simulink model "idq"  (R2021a)
settings: Solver=VariableStepAuto  StartTime=0.0  StopTime=0.2  FixedStep=1/150000  MaxStep=1e-6
undefined symbols (not defined in the file): in, ou
libraries: neural x105, spsMosfetLib x12, simulink x5, pid_lib x3, spsabctodq0Lib x3, spsFirstOrderFilterLib x2, spsPermanentMagnetSynchronousMachineLib x2, spsCurrentMeasurementLib x2, spsDCVoltageSourceLib x2, spsThreePhaseVIMeasurementLib x2, spsabctoAlphaBetaZeroLib x2, spsSVPWMGenerator2LevelLib x1
(part 4 of 7)

== system idq/NARX Neural Network - Closed Loop1/Layer 1/Delays 1 ==
  "p{1}" : Inport  PortDimensions=4  SampleTime=1e-05
      mask Display: e = 0.06;c1 = [120 230 180]/255;c2 = ([120 230 180]+0)/(256+128);c3 = ([120 230 180]+128)/(256+128);patch([0 1 1 0],[0 0 1 1],c1);patch([0 1 1 1-e 1-e 0+e],[0 0 1 1-e 0+e 0+e],c2);patch([0 0 1 1-e 0+e 0+e],[0 1 1 1-e 1-e 0+e],c3);plot([0 1 1 0 0],[0 0 1 1 0]);
  Delay 1 : UnitDelay  InitialCondition=pi_input_1_delayed_1  SampleTime=1e-05
      mask Display: e = 0.06;c1 = [120 150 230]/255;c2 = ([120 150 230]+0)/383;c3 = ([120 150 230]+128)/383;patch([0 1 1 0],[0 0 1 1],c1);patch([0 1 1 1-e 1-e 0+e],[0 0 1 1-e 0+e 0+e],c2);patch([0 0 1 1-e 0+e 0+e],[0 1 1 1-e 1-e 0+e],c3);plot([0 1 1 0 0],[0 0 1 1 0]);disp('D')
  Delay 10 : UnitDelay  InitialCondition=pi_input_1_delayed_10  SampleTime=1e-05
      mask Display: e = 0.06;c1 = [120 150 230]/255;c2 = ([120 150 230]+0)/383;c3 = ([120 150 230]+128)/383;patch([0 1 1 0],[0 0 1 1],c1);patch([0 1 1 1-e 1-e 0+e],[0 0 1 1-e 0+e 0+e],c2);patch([0 0 1 1-e 0+e 0+e],[0 1 1 1-e 1-e 0+e],c3);plot([0 1 1 0 0],[0 0 1 1 0]);disp('D')
  Delay 2 : UnitDelay  InitialCondition=pi_input_1_delayed_2  SampleTime=1e-05
      mask Display: e = 0.06;c1 = [120 150 230]/255;c2 = ([120 150 230]+0)/383;c3 = ([120 150 230]+128)/383;patch([0 1 1 0],[0 0 1 1],c1);patch([0 1 1 1-e 1-e 0+e],[0 0 1 1-e 0+e 0+e],c2);patch([0 0 1 1-e 0+e 0+e],[0 1 1 1-e 1-e 0+e],c3);plot([0 1 1 0 0],[0 0 1 1 0]);disp('D')
  Delay 3 : UnitDelay  InitialCondition=pi_input_1_delayed_3  SampleTime=1e-05
      mask Display: e = 0.06;c1 = [120 150 230]/255;c2 = ([120 150 230]+0)/383;c3 = ([120 150 230]+128)/383;patch([0 1 1 0],[0 0 1 1],c1);patch([0 1 1 1-e 1-e 0+e],[0 0 1 1-e 0+e 0+e],c2);patch([0 0 1 1-e 0+e 0+e],[0 1 1 1-e 1-e 0+e],c3);plot([0 1 1 0 0],[0 0 1 1 0]);disp('D')
  Delay 4 : UnitDelay  InitialCondition=pi_input_1_delayed_4  SampleTime=1e-05
      mask Display: e = 0.06;c1 = [120 150 230]/255;c2 = ([120 150 230]+0)/383;c3 = ([120 150 230]+128)/383;patch([0 1 1 0],[0 0 1 1],c1);patch([0 1 1 1-e 1-e 0+e],[0 0 1 1-e 0+e 0+e],c2);patch([0 0 1 1-e 0+e 0+e],[0 1 1 1-e 1-e 0+e],c3);plot([0 1 1 0 0],[0 0 1 1 0]);disp('D')
  Delay 5 : UnitDelay  InitialCondition=pi_input_1_delayed_5  SampleTime=1e-05
      mask Display: e = 0.06;c1 = [120 150 230]/255;c2 = ([120 150 230]+0)/383;c3 = ([120 150 230]+128)/383;patch([0 1 1 0],[0 0 1 1],c1);patch([0 1 1 1-e 1-e 0+e],[0 0 1 1-e 0+e 0+e],c2);patch([0 0 1 1-e 0+e 0+e],[0 1 1 1-e 1-e 0+e],c3);plot([0 1 1 0 0],[0 0 1 1 0]);disp('D')
  Delay 6 : UnitDelay  InitialCondition=pi_input_1_delayed_6  SampleTime=1e-05
      mask Display: e = 0.06;c1 = [120 150 230]/255;c2 = ([120 150 230]+0)/383;c3 = ([120 150 230]+128)/383;patch([0 1 1 0],[0 0 1 1],c1);patch([0 1 1 1-e 1-e 0+e],[0 0 1 1-e 0+e 0+e],c2);patch([0 0 1 1-e 0+e 0+e],[0 1 1 1-e 1-e 0+e],c3);plot([0 1 1 0 0],[0 0 1 1 0]);disp('D')
  Delay 7 : UnitDelay  InitialCondition=pi_input_1_delayed_7  SampleTime=1e-05
      mask Display: e = 0.06;c1 = [120 150 230]/255;c2 = ([120 150 230]+0)/383;c3 = ([120 150 230]+128)/383;patch([0 1 1 0],[0 0 1 1],c1);patch([0 1 1 1-e 1-e 0+e],[0 0 1 1-e 0+e 0+e],c2);patch([0 0 1 1-e 0+e 0+e],[0 1 1 1-e 1-e 0+e],c3);plot([0 1 1 0 0],[0 0 1 1 0]);disp('D')
  Delay 8 : UnitDelay  InitialCondition=pi_input_1_delayed_8  SampleTime=1e-05
      mask Display: e = 0.06;c1 = [120 150 230]/255;c2 = ([120 150 230]+0)/383;c3 = ([120 150 230]+128)/383;patch([0 1 1 0],[0 0 1 1],c1);patch([0 1 1 1-e 1-e 0+e],[0 0 1 1-e 0+e 0+e],c2);patch([0 0 1 1-e 0+e 0+e],[0 1 1 1-e 1-e 0+e],c3);plot([0 1 1 0 0],[0 0 1 1 0]);disp('D')
  Delay 9 : UnitDelay  InitialCondition=pi_input_1_delayed_9  SampleTime=1e-05
      mask Display: e = 0.06;c1 = [120 150 230]/255;c2 = ([120 150 230]+0)/383;c3 = ([120 150 230]+128)/383;patch([0 1 1 0],[0 0 1 1],c1);patch([0 1 1 1-e 1-e 0+e],[0 0 1 1-e 0+e 0+e],c2);patch([0 0 1 1-e 0+e 0+e],[0 1 1 1-e 1-e 0+e],c3);plot([0 1 1 0 0],[0 0 1 1 0]);disp('D')
  mux : Mux  Inputs=10
      mask Display: e = 0.06;c1 = [120 150 230]/255;c2 = ([120 150 230]+0)/383;c3 = ([120 150 230]+128)/383;patch([0 1 1 0],[0 0 1 1],c1);patch([0 1 1 1-e 1-e 0+e],[0 0 1 1-e 0+e 0+e],c2);patch([0 0 1 1-e 0+e 0+e],[0 1 1 1-e 1-e 0+e],c3);plot([0 1 1 0 0],[0 0 1 1 0]);disp('Mux')
  "pd{1,1}" : Outport
      mask Display: e = 0.06;c1 = [120 230 180]/255;c2 = ([120 230 180]+0)/(256+128);c3 = ([120 230 180]+128)/(256+128);patch([0 1 1 0],[0 0 1 1],c1);patch([0 1 1 1-e 1-e 0+e],[0 0 1 1-e 0+e 0+e],c2);patch([0 0 1 1-e 0+e 0+e],[0 1 1 1-e 1-e 0+e],c3);plot([0 1 1 0 0],[0 0 1 1 0]);
  wires:
  "p{1}"/1 -> Delay 1/1
  Delay 1/1 -> Delay 2/1, mux/1
  Delay 2/1 -> Delay 3/1, mux/2
  Delay 3/1 -> Delay 4/1, mux/3
  Delay 4/1 -> Delay 5/1, mux/4
  Delay 5/1 -> Delay 6/1, mux/5
  Delay 6/1 -> Delay 7/1, mux/6
  Delay 7/1 -> Delay 8/1, mux/7
  Delay 8/1 -> Delay 9/1, mux/8
  Delay 9/1 -> Delay 10/1, mux/9
  Delay 10/1 -> mux/10
  mux/1 -> "pd{1,1}"/1

== system idq/NARX Neural Network - Closed Loop1/Layer 1/Delays 2 ==
  "p{1}" : Inport  PortDimensions=1  SampleTime=1e-05
      mask Display: e = 0.06;c1 = [120 230 180]/255;c2 = ([120 230 180]+0)/(256+128);c3 = ([120 230 180]+128)/(256+128);patch([0 1 1 0],[0 0 1 1],c1);patch([0 1 1 1-e 1-e 0+e],[0 0 1 1-e 0+e 0+e],c2);patch([0 0 1 1-e 0+e 0+e],[0 1 1 1-e 1-e 0+e],c3);plot([0 1 1 0 0],[0 0 1 1 0]);
  Delay 1 : UnitDelay  InitialCondition=ai_layer_2_delayed_1  SampleTime=1e-05
      mask Display: e = 0.06;c1 = [120 150 230]/255;c2 = ([120 150 230]+0)/383;c3 = ([120 150 230]+128)/383;patch([0 1 1 0],[0 0 1 1],c1);patch([0 1 1 1-e 1-e 0+e],[0 0 1 1-e 0+e 0+e],c2);patch([0 0 1 1-e 0+e 0+e],[0 1 1 1-e 1-e 0+e],c3);plot([0 1 1 0 0],[0 0 1 1 0]);disp('D')
  Delay 10 : UnitDelay  InitialCondition=ai_layer_2_delayed_10  SampleTime=1e-05
      mask Display: e = 0.06;c1 = [120 150 230]/255;c2 = ([120 150 230]+0)/383;c3 = ([120 150 230]+128)/383;patch([0 1 1 0],[0 0 1 1],c1);patch([0 1 1 1-e 1-e 0+e],[0 0 1 1-e 0+e 0+e],c2);patch([0 0 1 1-e 0+e 0+e],[0 1 1 1-e 1-e 0+e],c3);plot([0 1 1 0 0],[0 0 1 1 0]);disp('D')
  Delay 2 : UnitDelay  InitialCondition=ai_layer_2_delayed_2  SampleTime=1e-05
      mask Display: e = 0.06;c1 = [120 150 230]/255;c2 = ([120 150 230]+0)/383;c3 = ([120 150 230]+128)/383;patch([0 1 1 0],[0 0 1 1],c1);patch([0 1 1 1-e 1-e 0+e],[0 0 1 1-e 0+e 0+e],c2);patch([0 0 1 1-e 0+e 0+e],[0 1 1 1-e 1-e 0+e],c3);plot([0 1 1 0 0],[0 0 1 1 0]);disp('D')
  Delay 3 : UnitDelay  InitialCondition=ai_layer_2_delayed_3  SampleTime=1e-05
      mask Display: e = 0.06;c1 = [120 150 230]/255;c2 = ([120 150 230]+0)/383;c3 = ([120 150 230]+128)/383;patch([0 1 1 0],[0 0 1 1],c1);patch([0 1 1 1-e 1-e 0+e],[0 0 1 1-e 0+e 0+e],c2);patch([0 0 1 1-e 0+e 0+e],[0 1 1 1-e 1-e 0+e],c3);plot([0 1 1 0 0],[0 0 1 1 0]);disp('D')
  Delay 4 : UnitDelay  InitialCondition=ai_layer_2_delayed_4  SampleTime=1e-05
      mask Display: e = 0.06;c1 = [120 150 230]/255;c2 = ([120 150 230]+0)/383;c3 = ([120 150 230]+128)/383;patch([0 1 1 0],[0 0 1 1],c1);patch([0 1 1 1-e 1-e 0+e],[0 0 1 1-e 0+e 0+e],c2);patch([0 0 1 1-e 0+e 0+e],[0 1 1 1-e 1-e 0+e],c3);plot([0 1 1 0 0],[0 0 1 1 0]);disp('D')
  Delay 5 : UnitDelay  InitialCondition=ai_layer_2_delayed_5  SampleTime=1e-05
      mask Display: e = 0.06;c1 = [120 150 230]/255;c2 = ([120 150 230]+0)/383;c3 = ([120 150 230]+128)/383;patch([0 1 1 0],[0 0 1 1],c1);patch([0 1 1 1-e 1-e 0+e],[0 0 1 1-e 0+e 0+e],c2);patch([0 0 1 1-e 0+e 0+e],[0 1 1 1-e 1-e 0+e],c3);plot([0 1 1 0 0],[0 0 1 1 0]);disp('D')
  Delay 6 : UnitDelay  InitialCondition=ai_layer_2_delayed_6  SampleTime=1e-05
      mask Display: e = 0.06;c1 = [120 150 230]/255;c2 = ([120 150 230]+0)/383;c3 = ([120 150 230]+128)/383;patch([0 1 1 0],[0 0 1 1],c1);patch([0 1 1 1-e 1-e 0+e],[0 0 1 1-e 0+e 0+e],c2);patch([0 0 1 1-e 0+e 0+e],[0 1 1 1-e 1-e 0+e],c3);plot([0 1 1 0 0],[0 0 1 1 0]);disp('D')
  Delay 7 : UnitDelay  InitialCondition=ai_layer_2_delayed_7  SampleTime=1e-05
      mask Display: e = 0.06;c1 = [120 150 230]/255;c2 = ([120 150 230]+0)/383;c3 = ([120 150 230]+128)/383;patch([0 1 1 0],[0 0 1 1],c1);patch([0 1 1 1-e 1-e 0+e],[0 0 1 1-e 0+e 0+e],c2);patch([0 0 1 1-e 0+e 0+e],[0 1 1 1-e 1-e 0+e],c3);plot([0 1 1 0 0],[0 0 1 1 0]);disp('D')
  Delay 8 : UnitDelay  InitialCondition=ai_layer_2_delayed_8  SampleTime=1e-05
      mask Display: e = 0.06;c1 = [120 150 230]/255;c2 = ([120 150 230]+0)/383;c3 = ([120 150 230]+128)/383;patch([0 1 1 0],[0 0 1 1],c1);patch([0 1 1 1-e 1-e 0+e],[0 0 1 1-e 0+e 0+e],c2);patch([0 0 1 1-e 0+e 0+e],[0 1 1 1-e 1-e 0+e],c3);plot([0 1 1 0 0],[0 0 1 1 0]);disp('D')
  Delay 9 : UnitDelay  InitialCondition=ai_layer_2_delayed_9  SampleTime=1e-05
      mask Display: e = 0.06;c1 = [120 150 230]/255;c2 = ([120 150 230]+0)/383;c3 = ([120 150 230]+128)/383;patch([0 1 1 0],[0 0 1 1],c1);patch([0 1 1 1-e 1-e 0+e],[0 0 1 1-e 0+e 0+e],c2);patch([0 0 1 1-e 0+e 0+e],[0 1 1 1-e 1-e 0+e],c3);plot([0 1 1 0 0],[0 0 1 1 0]);disp('D')
  mux : Mux  Inputs=10
      mask Display: e = 0.06;c1 = [120 150 230]/255;c2 = ([120 150 230]+0)/383;c3 = ([120 150 230]+128)/383;patch([0 1 1 0],[0 0 1 1],c1);patch([0 1 1 1-e 1-e 0+e],[0 0 1 1-e 0+e 0+e],c2);patch([0 0 1 1-e 0+e 0+e],[0 1 1 1-e 1-e 0+e],c3);plot([0 1 1 0 0],[0 0 1 1 0]);disp('Mux')
  "pd{1,2}" : Outport
      mask Display: e = 0.06;c1 = [120 230 180]/255;c2 = ([120 230 180]+0)/(256+128);c3 = ([120 230 180]+128)/(256+128);patch([0 1 1 0],[0 0 1 1],c1);patch([0 1 1 1-e 1-e 0+e],[0 0 1 1-e 0+e 0+e],c2);patch([0 0 1 1-e 0+e 0+e],[0 1 1 1-e 1-e 0+e],c3);plot([0 1 1 0 0],[0 0 1 1 0]);
  wires:
  "p{1}"/1 -> Delay 1/1
  Delay 1/1 -> Delay 2/1, mux/1
  Delay 2/1 -> Delay 3/1, mux/2
  Delay 3/1 -> Delay 4/1, mux/3
  Delay 4/1 -> Delay 5/1, mux/4
  Delay 5/1 -> Delay 6/1, mux/5
  Delay 6/1 -> Delay 7/1, mux/6
  Delay 7/1 -> Delay 8/1, mux/7
  Delay 8/1 -> Delay 9/1, mux/8
  Delay 9/1 -> Delay 10/1, mux/9
  Delay 10/1 -> mux/10
  mux/1 -> "pd{1,2}"/1

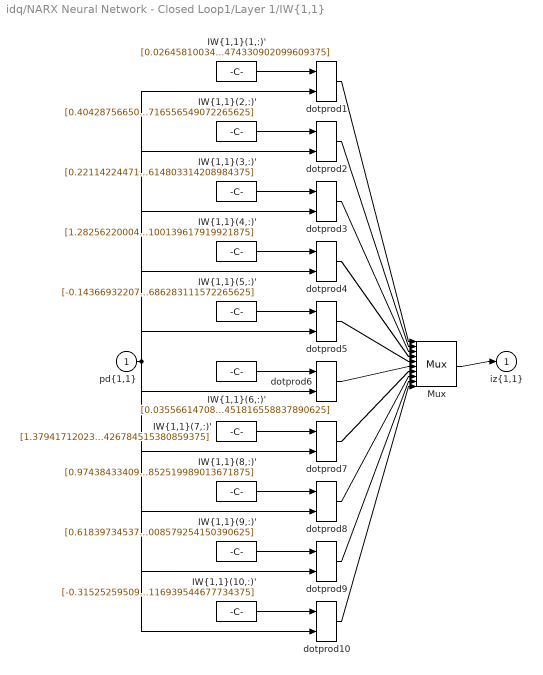
== system idq/NARX Neural Network - Closed Loop1/Layer 1/IW{1,1} ==
  "pd{1,1}" : Inport  PortDimensions=40  SampleTime=1e-05
      mask Display: e = 0.06;c1 = [120 230 180]/255;c2 = ([120 230 180]+0)/(256+128);c3 = ([120 230 180]+128)/(256+128);patch([0 1 1 0],[0 0 1 1],c1);patch([0 1 1 1-e 1-e 0+e],[0 0 1 1-e 0+e 0+e],c2);patch([0 0 1 1-e 0+e 0+e],[0 1 1 1-e 1-e 0+e],c3);plot([0 1 1 0 0],[0 0 1 1 0]);
  "IW{1,1}(1,:)'" : Constant  Value=[0.0264581003444631403243025857818793156184256076812744140625;-0.155011872361149716237349593939143233001232147216796875;0.2800450015320554708608824512339197099208831787109375;-0.035999332393767770332804190047681913711130619049072265625;-0.0231031095312188294865762827612343244254589080810546875;-0.01084188405027063963059763551655123592354357242584228515625;0.2257599227818586073990303475511609576642513275146484375;-0.01362265239200942390507265145060955546796321868896484375;0.0032402507072451232177090485464532321202568709850311279296875;0.0441032571786067195684921671272604726254940032958984375;0.165701195358703701199232227736501954495906829833984375;0.007809907479812143622777131923839988303370773792266845703125;-0.32247695162340495045327770640142261981964111328125;0.05464320885084562873235114466297090984880924224853515625;0.11734475609666546180864798998300102539360523223876953125;0.022042370696496817183973604414859437383711338043212890625;-0.14779113146788847021895207944908179342746734619140625;-0.04890170810500689413391484094972838647663593292236328125;0.06125385435683612656010410546514322049915790557861328125;0.04759689912071306261420744476708932779729366302490234375;-0.15368472929600895948709649019292555749416351318359375;-0.0281595220718017270888910985604525194503366947174072265625;0.0018987226084477061040234335820287014939822256565093994140625;0.073658755859801861021196600631810724735260009765625;-0.4288729543974467706135555999935604631900787353515625;0.08828076784965165069163361977189197205007076263427734375;-0.050871065802078618833803602683474309742450714111328125;0.0882362530759153440573783200306934304535388946533203125;-0.1793763053182588496081706352924811653792858123779296875;0.07017420686064583523755544547384488396346569061279296875;-0.117282277187744810031944098227540962398052215576171875;0.11202104378384718230687866480366210453212261199951171875;-0.25554474369071378259121729570324532687664031982421875;0.027017848729185854617096396168562932871282100677490234375;-0.1817393554574067149331995096872560679912567138671875;0.1373281770518507693967791283284896053373813629150390625;-0.204404914050620833965155043188133276998996734619140625;-0.0668232496942136877660090021890937350690364837646484375;-0.24882893572699382733759421171271242201328277587890625;0.1701278181676374179343014247933751903474330902099609375]
      mask Display: e = 0.06;c1 = [120 150 230]/255;c2 = ([120 150 230]+0)/383;c3 = ([120 150 230]+128)/383;patch([0 1 1 0],[0 0 1 1],c1);patch([0 1 1 1-e 1-e 0+e],[0 0 1 1-e 0+e 0+e],c2);patch([0 0 1 1-e 0+e 0+e],[0 1 1 1-e 1-e 0+e],c3);plot([0 1 1 0 0],[0 0 1 1 0]);disp('Weights');
  "IW{1,1}(10,:)'" : Constant  Value=[-0.31525259509166925209200371682527475059032440185546875;0.031430264941845940940279291453407495282590389251708984375;0.04300350121840725015065487468746141530573368072509765625;0.104894086313607914906498308482696302235126495361328125;-0.1566655845537998914540622763524879701435565948486328125;-0.0716047747138739698602449834652361460030078887939453125;0.03605058399281184378093456643910030834376811981201171875;0.099112432287408680497975410617073066532611846923828125;-0.0631150029612531915379491920248256064951419830322265625;-0.0043770460200082093871198907208963646553456783294677734375;0.0244605474216665376430146494612927199341356754302978515625;0.09132734885736548680057467208825983107089996337890625;0.207052989213431792858699509451980702579021453857421875;-0.0228252538418006155340744811610420583747327327728271484375;0.0028134491170567327809892699264082693844102323055267333984375;0.0912201671514198952905871919938363134860992431640625;-0.04176167714776944650534318270729272626340389251708984375;0.044189429996556554847142450626051868312060832977294921875;-0.00765293292163178075215856921431623050011694431304931640625;0.07987739077519741270894115814371616579592227935791015625;-0.331119784378241188704805608722381293773651123046875;0.0302182814086223404392850255817393190227448940277099609375;-0.0024997052890350555075238414559635202749632298946380615234375;0.06064491989298048668644014469464309513568878173828125;-0.09372638971693357523573553180540329776704311370849609375;-0.08371495819516942826776784158937516622245311737060546875;-0.0029028284625321628363570081177158499485813081264495849609375;0.0520617771870836854031239226969773881137371063232421875;-0.391090681424232922136496881648781709372997283935546875;-0.00136907171975723072898656340612433268688619136810302734375;0.00956503245403937142621320077751079224981367588043212890625;0.0307965875047167721156871067478277836926281452178955078125;-0.16791018620316766618572046354529447853565216064453125;0.052104895448455000595000541352419531904160976409912109375;0.01218678401046962948839347262719456921331584453582763671875;0.0115547261342168229580895655317362979985773563385009765625;-0.28622811444357931787152438118937425315380096435546875;0.070737838842561184815593833263847045600414276123046875;0.0215860086936635504895054538110343855805695056915283203125;-0.01312540017539457447293127501097842468880116939544677734375]
      mask Display: e = 0.06;c1 = [120 150 230]/255;c2 = ([120 150 230]+0)/383;c3 = ([120 150 230]+128)/383;patch([0 1 1 0],[0 0 1 1],c1);patch([0 1 1 1-e 1-e 0+e],[0 0 1 1-e 0+e 0+e],c2);patch([0 0 1 1-e 0+e 0+e],[0 1 1 1-e 1-e 0+e],c3);plot([0 1 1 0 0],[0 0 1 1 0]);disp('Weights');
  "IW{1,1}(2,:)'" : Constant  Value=[0.404287566502792572453728325854171998798847198486328125;-0.403250328667407564875446723817731253802776336669921875;-0.14999270628009586658890839316882193088531494140625;-0.10364376733671888664023441606332198716700077056884765625;0.2307448742481465198128631755025708116590976715087890625;-0.050437412703318300344346170049902866594493389129638671875;-0.1268057176436730160151711288563092239201068878173828125;-0.0735196425771490191802826075218035839498043060302734375;0.0312264234689138171774391850021856953389942646026611328125;0.025309091997740999768762293342660996131598949432373046875;-0.09863467125859355644212911329304915852844715118408203125;-0.04998643840051801567891942568166996352374553680419921875;0.0006075840790996903280352103848827027832157909870147705078125;0.2392835782778407194282266345908283255994319915771484375;-0.0768766146018567686493128121583140455186367034912109375;-0.03444269992289779314109665619980660267174243927001953125;-0.1219129140038336667206664287732564844191074371337890625;0.2146381724825902337361327454345882870256900787353515625;-0.05051196470921050230007409709287458099424839019775390625;-0.018469912687682756013973772724057198502123355865478515625;-0.039545617926555483301331861412108992226421833038330078125;0.0839823188821113841839860469917766749858856201171875;-0.0261787150990239574077644846283874358050525188446044921875;0.00931515752711300527855176056846175924874842166900634765625;-0.09378701116329817011330050036121974699199199676513671875;0.1352867271855986708306573973459308035671710968017578125;-0.002328895548274922087939042825155411264859139919281005859375;0.03612202944687463446182817961016553454101085662841796875;-0.045450745297773757769288494046122650615870952606201171875;0.10946810546046414902576771055464632809162139892578125;0.01812079419329916396552704327405081130564212799072265625;0.06810342611095783482699772548585315234959125518798828125;0.021846413108170710526412250374050927348434925079345703125;0.039722976835466890233039549684690427966415882110595703125;0.03589736716743642530591529293815256096422672271728515625;0.10879854600166682931927653044112958014011383056640625;0.27192689385129475976299318062956444919109344482421875;-0.0904090904617108337415487540056346915662288665771484375;0.044637242455090216097790545290990849025547504425048828125;0.165454465081222912292702176273451186716556549072265625]
      mask Display: e = 0.06;c1 = [120 150 230]/255;c2 = ([120 150 230]+0)/383;c3 = ([120 150 230]+128)/383;patch([0 1 1 0],[0 0 1 1],c1);patch([0 1 1 1-e 1-e 0+e],[0 0 1 1-e 0+e 0+e],c2);patch([0 0 1 1-e 0+e 0+e],[0 1 1 1-e 1-e 0+e],c3);plot([0 1 1 0 0],[0 0 1 1 0]);disp('Weights');
  "IW{1,1}(3,:)'" : Constant  Value=[0.221142244717192515413017872560885734856128692626953125;-0.93569778660913660583986484198248945176601409912109375;-1.18193435088941267707696169964037835597991943359375;-0.0576548752107831907753876521383062936365604400634765625;-0.083464223785847224679201872277189977467060089111328125;0.2316834866348068400210280515238991938531398773193359375;-0.90330499677291964388814449193887412548065185546875;-0.07798091210921719029780518894767737947404384613037109375;-0.038333916777752129190215413245823583565652370452880859375;0.39234373433914970785707510003703646361827850341796875;-0.6371763488163775246420073017361573874950408935546875;-0.0965804397690620819449947020984836854040622711181640625;0.07228590763652760486923654070778866298496723175048828125;0.233456318481962465938295281375758349895477294921875;-0.377851239329094978902645607377053238451480865478515625;-0.09594709433470365034235527446071500889956951141357421875;0.173287318955856528557291085235192440450191497802734375;-0.06467152694635820708857210092901368625462055206298828125;-0.1208347215062860746659367805477813817560672760009765625;-0.0691736180452788562700305874386685900390148162841796875;0.303046772479661774557513354011462070047855377197265625;0.01972742994564956331426941460449597798287868499755859375;0.12176082911210799053502995548114995472133159637451171875;-0.033168749645479535248515645662337192334234714508056640625;0.003865938247603996520684876969653487321920692920684814453125;0.34681971256624333221907363622449338436126708984375;0.36326053562087057269280876425909809768199920654296875;-0.011798579347776984305173897382701397873461246490478515625;0.148265515962799743210354108668980188667774200439453125;0.057579935576568604116420857508273911662399768829345703125;0.60030762805748205668265882195555604994297027587890625;0.0370669086746271692067722369756666012108325958251953125;0.072827707977203004485744486373732797801494598388671875;0.0954199738374567896226352559096994809806346893310546875;0.83437310038273737600178492357372306287288665771484375;0.0913851205560543833339437469476251862943172454833984375;-0.01373924844856483189203810724166032741777598857879638671875;0.0665529738372798440604327652181382291018962860107421875;1.0682475405566993487127547268755733966827392578125;0.1546512514275143190811689919428317807614803314208984375]
      mask Display: e = 0.06;c1 = [120 150 230]/255;c2 = ([120 150 230]+0)/383;c3 = ([120 150 230]+128)/383;patch([0 1 1 0],[0 0 1 1],c1);patch([0 1 1 1-e 1-e 0+e],[0 0 1 1-e 0+e 0+e],c2);patch([0 0 1 1-e 0+e 0+e],[0 1 1 1-e 1-e 0+e],c3);plot([0 1 1 0 0],[0 0 1 1 0]);disp('Weights');
  "IW{1,1}(4,:)'" : Constant  Value=[1.2825622000457881366486390106729231774806976318359375;0.6402270753918768431134367347112856805324554443359375;0.53364884910127596828743890000623650848865509033203125;0.96199324746704295563404230051673948764801025390625;-0.139261364653506358735057801823131740093231201171875;-0.260514823449439159031015833534183911979198455810546875;0.394949614591090014670271557406522333621978759765625;0.77048498608680071608745265621109865605831146240234375;-0.265109506085548840559340533218346536159515380859375;-0.056944306762786216224991875378691474907100200653076171875;0.26531667436419581473927564729820005595684051513671875;0.5605775243995976264699265811941586434841156005859375;-0.459430370835424095599108795795473270118236541748046875;-0.373647780412811714167986565371393226087093353271484375;0.16332127347459224342429706666735000908374786376953125;0.355512911319332436388407359117991290986537933349609375;0.1961768610027908865678369920715340413153171539306640625;-0.0199481518591114494187710448613870539702475070953369140625;0.030391735428321443868160400825217948295176029205322265625;0.145156359393597778062456882253172807395458221435546875;-0.025821863709085034199741670590810826979577541351318359375;-0.323311266568750033112422670455998741090297698974609375;-0.074091974567163709775030611126567237079143524169921875;-0.06210378401063700037898485106779844500124454498291015625;-0.258294007728911534371718516922555863857269287109375;-0.4337132989973355723378745096852071583271026611328125;-0.1548377192350678666077357092945021577179431915283203125;-0.276005961790680320877555686820414848625659942626953125;0.0853071013728281257737506848570774309337139129638671875;-0.01268666256750173963741001870175750809721648693084716796875;-0.253654816395552595853501998135470785200595855712890625;-0.50749597275972313514813549772952683269977569580078125;0.0974932477928580620840648407465778291225433349609375;-0.00628293356560590855741654792154804454185068607330322265625;-0.34338210644061184506625750145758502185344696044921875;-0.745017980219321085399997173226438462734222412109375;-0.033180049462065312748659806629802915267646312713623046875;-0.109708109101965212150986417327658273279666900634765625;-0.414738719536782818320119758936925791203975677490234375;-0.98713307347126011404014889194513671100139617919921875]
      mask Display: e = 0.06;c1 = [120 150 230]/255;c2 = ([120 150 230]+0)/383;c3 = ([120 150 230]+128)/383;patch([0 1 1 0],[0 0 1 1],c1);patch([0 1 1 1-e 1-e 0+e],[0 0 1 1-e 0+e 0+e],c2);patch([0 0 1 1-e 0+e 0+e],[0 1 1 1-e 1-e 0+e],c3);plot([0 1 1 0 0],[0 0 1 1 0]);disp('Weights');
  "IW{1,1}(5,:)'" : Constant  Value=[-0.1436693220731536657641669307849952019751071929931640625;-0.52115555265366031445495309526450000703334808349609375;0.456837527095214801509115432054386474192142486572265625;0.242177332460095484645279384494642727077007293701171875;-0.038548067158590874903278944429985131137073040008544921875;0.097331656080749284765119000439881347119808197021484375;0.374041633215228319642164933611638844013214111328125;0.185228038407303008394677590331411920487880706787109375;-0.08123835698259425364131658398036961443722248077392578125;0.077775369477721179034546139519079588353633880615234375;0.289649153566691908157082480101962573826313018798828125;0.1292714841253526369957427277768147177994251251220703125;-0.01497618847007181445973866829035614500753581523895263671875;-0.05580311822230864249316795167032978497445583343505859375;0.201764684459868559596174009129754267632961273193359375;0.08309633418715101083051877139951102435588836669921875;-0.0728106788515201219791350695231813006103038787841796875;-0.0938938294456459210390875114171649329364299774169921875;0.11309155542180006348562670837054611183702945709228515625;0.038978398558627336267790042256820015609264373779296875;0.1293630264530249152077345797806628979742527008056640625;-0.130215304673179266270466314381337724626064300537109375;0.01237366003115742026097212402646619011647999286651611328125;0.0036234483096465237329797393073249622830189764499664306640625;0.10966413902600401220066572705036378465592861175537109375;-0.1544650141417591715509161076624877750873565673828125;-0.0915698308528863635924466279902844689786434173583984375;-0.029221939429442504720935147588534164242446422576904296875;0.055667093575187905074574956643118639476597309112548828125;-0.1283673098737740103647553269183845259249210357666015625;-0.197545396603328260454190967720933258533477783203125;-0.062766192488151906214710606946027837693691253662109375;0.01455338426129008065623704482050015940330922603607177734375;0.0210914406915475062531672989507569582201540470123291015625;-0.3105121782189390611250701113021932542324066162109375;-0.10291752901469695957725747348376899026334285736083984375;-0.1895138041201333833907227699455688707530498504638671875;-0.012199939972507234386966956662945449352264404296875;-0.41695785435362575643836180461221374571323394775390625;-0.1456274279498782908692788851112709380686283111572265625]
      mask Display: e = 0.06;c1 = [120 150 230]/255;c2 = ([120 150 230]+0)/383;c3 = ([120 150 230]+128)/383;patch([0 1 1 0],[0 0 1 1],c1);patch([0 1 1 1-e 1-e 0+e],[0 0 1 1-e 0+e 0+e],c2);patch([0 0 1 1-e 0+e 0+e],[0 1 1 1-e 1-e 0+e],c3);plot([0 1 1 0 0],[0 0 1 1 0]);disp('Weights');
  "IW{1,1}(6,:)'" : Constant  Value=[0.035566147080295644478109551300804014317691326141357421875;1.345785589579339358579090912826359272003173828125;-0.402906207477657096749368292876170016825199127197265625;0.6797986720358419887588752317242324352264404296875;0.1369844627955762172977216550862067379057407379150390625;-0.244618091905704992949921461331541649997234344482421875;-0.318939589811643442462951725246966816484928131103515625;0.5468220724001309207551457802765071392059326171875;-0.10129533944925443733620085140501032583415508270263671875;-0.1906079832647604443973676779933157376945018768310546875;-0.224199234750296738649666394849191419780254364013671875;0.400797496245371143164248906032298691570758819580078125;0.194530764469177663844590142616652883589267730712890625;-0.484814007758827714145155596270342357456684112548828125;-0.1335829358782410214434577255815383978188037872314453125;0.273897227163087675361197170786908827722072601318359375;0.08667904927128806946701189417581190355122089385986328125;0.1450573233288394714435298737953417003154754638671875;-0.053656940684528871277070294354416546411812305450439453125;0.10934734467499594712247557026785216294229030609130859375;-0.00066320457097665693434185296695204669958911836147308349609375;-0.17630078494639878083916073592263273894786834716796875;0.041018036895985064693714861050466424785554409027099609375;-0.04562004192104786304273744690362946130335330963134765625;0.1764386046788267992102561265710392035543918609619140625;-0.34122065016222913325094623360200785100460052490234375;0.133543882194234464488857838659896515309810638427734375;-0.1914562069350406459111724188915104605257511138916015625;0.12449080008476608172340860392068861983716487884521484375;0.0713948797367921772494270271636196412146091461181640625;0.219164746054576642375621986502665095031261444091796875;-0.362862091309917644821325666271150112152099609375;0.05680601033967312696315588027573539875447750091552734375;-0.15032042761891550863850852692849002778530120849609375;0.316045041099419943275705691121402196586132049560546875;-0.52882727105184923477310121597838588058948516845703125;0.039591312184570272292294390581446350552141666412353515625;-0.006793897015509945021272120158073448692448437213897705078125;0.4117040028798018003186598434695042669773101806640625;-0.7069369862728311915134327136911451816558837890625]
      mask Display: e = 0.06;c1 = [120 150 230]/255;c2 = ([120 150 230]+0)/383;c3 = ([120 150 230]+128)/383;patch([0 1 1 0],[0 0 1 1],c1);patch([0 1 1 1-e 1-e 0+e],[0 0 1 1-e 0+e 0+e],c2);patch([0 0 1 1-e 0+e 0+e],[0 1 1 1-e 1-e 0+e],c3);plot([0 1 1 0 0],[0 0 1 1 0]);disp('Weights');
  "IW{1,1}(7,:)'" : Constant  Value=[1.3794171202312257573652232167660258710384368896484375;-0.346159581390041548587532815872691571712493896484375;-0.280179859204263859151495807964238338172435760498046875;-0.98385897765413010684909522751695476472377777099609375;-0.2003186301421425452584657023180625401437282562255859375;0.156900467902397144914772297852323390543460845947265625;-0.22906869957036024576524368967511691153049468994140625;-0.78775001312269277153887969689094461500644683837890625;-0.38174267080154777875833360667456872761249542236328125;0.1324864654721847057050609919315320439636707305908203125;-0.16405012415898301281202975587802939116954803466796875;-0.58785346579363562113940133713185787200927734375;-0.167994405456998341374941219328320585191249847412109375;0.176292723392869887799605521649937145411968231201171875;-0.1045829654285750642817021116570685990154743194580078125;-0.37749848443712508139213923641364090144634246826171875;0.082772773035674596098232314034248702228069305419921875;0.1294183070281687275571158579623443074524402618408203125;-0.0503420361205701993867478449828922748565673828125;-0.1504635381740809518813506429069093428552150726318359375;-0.100037971533307568083870364716858603060245513916015625;0.329756241550632267500731131804059259593486785888671875;0.0116518794676253763242801397836956311948597431182861328125;0.0689387221945856054627910225462983362376689910888671875;-0.367657730501671498046789565705694258213043212890625;0.199258844350138686341011862168670631945133209228515625;0.0948296532709312078868180151403066702187061309814453125;0.295389495378936828284821558554540388286113739013671875;0.1463406226896686590510654468744178302586078643798828125;0.168389726960378849351940289125195704400539398193359375;0.1604769393953356104720597841151175089180469512939453125;0.54434379618925288202291312700253911316394805908203125;-0.068339219469893575098495830388856120407581329345703125;-0.000101575569080491513729302965884926379658281803131103515625;0.2459985141047987544649089386439300142228603363037109375;0.80413412753415680622737227167817763984203338623046875;0.062828711586723373638818657127558253705501556396484375;0.0688712031143426106627458693765220232307910919189453125;0.329053990697458498271288362957420758903026580810546875;1.0719995747386759088470853384933434426784515380859375]
      mask Display: e = 0.06;c1 = [120 150 230]/255;c2 = ([120 150 230]+0)/383;c3 = ([120 150 230]+128)/383;patch([0 1 1 0],[0 0 1 1],c1);patch([0 1 1 1-e 1-e 0+e],[0 0 1 1-e 0+e 0+e],c2);patch([0 0 1 1-e 0+e 0+e],[0 1 1 1-e 1-e 0+e],c3);plot([0 1 1 0 0],[0 0 1 1 0]);disp('Weights');
  "IW{1,1}(8,:)'" : Constant  Value=[0.97438433409955849118233572880853898823261260986328125;-0.50390909693759977638904956620535813271999359130859375;1.1406444943419000725981504729134030640125274658203125;0.1935714233930634076141785726576927118003368377685546875;-0.230037626477283596582168456734507344663143157958984375;-0.076736593426837196307843669274006970226764678955078125;0.91019517772409452849302624599658884108066558837890625;0.1321891942940303377174160459617269225418567657470703125;-0.293801308204964806147785338907851837575435638427734375;0.067087200562759463640105650483747012913227081298828125;0.6731804084951900080113773583434522151947021484375;0.06894127180237485941205477502080611884593963623046875;-0.300343618894015562670318786331336013972759246826171875;0.0293728393451675728886840488485177047550678253173828125;0.432317865112309906994170205507543869316577911376953125;0.014196811312635525259562285782521939836442470550537109375;0.10574480566003581494260998852041666395962238311767578125;-0.2305338633778089285630841231977683492004871368408203125;0.1737485146974411531761717242261511273682117462158203125;-0.0102633279302546502609327916388792800717055797576904296875;-0.4540161760713943284173410575021989643573760986328125;0.1341797762717078512650914490222930908203125;-0.0747769471183115097545623939367942512035369873046875;-0.060102155936104163791444676689934567548334598541259765625;-0.34702650629720255270882489639916457235813140869140625;-0.1034035988974625619452041291879140771925449371337890625;-0.326907571920222628225616290364996530115604400634765625;-0.08885647364366595912787971656143781729042530059814453125;-0.0354193541146306800637688638744293712079524993896484375;-0.06495838795744911242646679738754755817353725433349609375;-0.60027914743814958509204871006659232079982757568359375;-0.10432799258671097974993102752705453895032405853271484375;-0.08321176893842792410271869130156119354069232940673828125;-0.1610280895387994071210613356015528552234172821044921875;-0.8744657426783837284034461845294572412967681884765625;-0.10896657652523010495482225223895511589944362640380859375;-0.04725140985798427506470176240327418781816959381103515625;0.00588466871349959362580417376875629997812211513519287109375;-1.1602171879175264823658153545693494379520416259765625;-0.113467461566041094567225400169263593852519989013671875]
      mask Display: e = 0.06;c1 = [120 150 230]/255;c2 = ([120 150 230]+0)/383;c3 = ([120 150 230]+128)/383;patch([0 1 1 0],[0 0 1 1],c1);patch([0 1 1 1-e 1-e 0+e],[0 0 1 1-e 0+e 0+e],c2);patch([0 0 1 1-e 0+e 0+e],[0 1 1 1-e 1-e 0+e],c3);plot([0 1 1 0 0],[0 0 1 1 0]);disp('Weights');
  "IW{1,1}(9,:)'" : Constant  Value=[0.6183973453739375347737450283602811396121978759765625;1.09712775640001058974348779884167015552520751953125;0.5366859997957134087442909731180407106876373291015625;-0.7033911209318663981804320428636856377124786376953125;-0.22148016560278749320644919862388633191585540771484375;-0.0493755413216548089128110632373136468231678009033203125;0.41313742358017491174138058340759016573429107666015625;-0.5750293827005032998300748658948577940464019775390625;-0.14586096829948258513098835464916191995143890380859375;-0.335605340685345365780989368431619368493556976318359375;0.2975482081534004397127546326373703777790069580078125;-0.422489371354158815830004414237919263541698455810546875;-0.318728383934667791610451104133971966803073883056640625;-0.1484889040812145122316678680363111197948455810546875;0.188557831206639547882986107651959173381328582763671875;-0.27562342932120309502153077119146473705768585205078125;0.00792415563835606288900503813010800513438880443572998046875;0.1634749328335560469849241371775860898196697235107421875;0.058922429004700883903300479005338274873793125152587890625;-0.1269568559563718224136863454987178556621074676513671875;-0.1410031922517243907488904142155661247670650482177734375;0.023565755460954129762995989949558861553668975830078125;-0.0561746286176641185239333253775839693844318389892578125;0.032333057226810180129206173660350032150745391845703125;-0.304173061325831051160406559574767015874385833740234375;-0.1393205849683144259554268273859634064137935638427734375;-0.1556257721937459315153517991348053328692913055419921875;0.20408972540137437778895446172100491821765899658203125;-0.08098224483692784136934506022953428328037261962890625;-0.05134656823816539927829438738626777194440364837646484375;-0.263867962261181532301890229064156301319599151611328125;0.38537728736803089635287733472068794071674346923828125;-0.057753154616932013409869028919274569489061832427978515625;0.1476803056217402543293104599797516129910945892333984375;-0.37505050817680862795810980969690717756748199462890625;0.56543857536013664155660762844490818679332733154296875;-0.1054480317913007725305618578204303048551082611083984375;0.047941739282653154929914052218009601347148418426513671875;-0.477021505780948318342638003741740249097347259521484375;0.75796026157484386320817293380969204008579254150390625]
      mask Display: e = 0.06;c1 = [120 150 230]/255;c2 = ([120 150 230]+0)/383;c3 = ([120 150 230]+128)/383;patch([0 1 1 0],[0 0 1 1],c1);patch([0 1 1 1-e 1-e 0+e],[0 0 1 1-e 0+e 0+e],c2);patch([0 0 1 1-e 0+e 0+e],[0 1 1 1-e 1-e 0+e],c3);plot([0 1 1 0 0],[0 0 1 1 0]);disp('Weights');
  Mux : Mux  Inputs=10
      mask Display: e = 0.06;c1 = [120 150 230]/255;c2 = ([120 150 230]+0)/383;c3 = ([120 150 230]+128)/383;patch([0 1 1 0],[0 0 1 1],c1);patch([0 1 1 1-e 1-e 0+e],[0 0 1 1-e 0+e 0+e],c2);patch([0 0 1 1-e 0+e 0+e],[0 1 1 1-e 1-e 0+e],c3);plot([0 1 1 0 0],[0 0 1 1 0]);disp('Mux');
  dotprod{1..10} (10 alike) : neural/Weight Functions/dotprod
  "iz{1,1}" : Outport
      mask Display: e = 0.06;c1 = [120 230 180]/255;c2 = ([120 230 180]+0)/(256+128);c3 = ([120 230 180]+128)/(256+128);patch([0 1 1 0],[0 0 1 1],c1);patch([0 1 1 1-e 1-e 0+e],[0 0 1 1-e 0+e 0+e],c2);patch([0 0 1 1-e 0+e 0+e],[0 1 1 1-e 1-e 0+e],c3);plot([0 1 1 0 0],[0 0 1 1 0]);
  wires:
  "IW{1,1}(1,:)'"/1 -> dotprod1/1
  "pd{1,1}"/1 -> dotprod1/2, dotprod2/2, dotprod3/2, dotprod4/2, dotprod5/2, dotprod6/2, dotprod7/2, dotprod8/2, dotprod9/2, dotprod10/2
  dotprod1/1 -> Mux/1
  "IW{1,1}(2,:)'"/1 -> dotprod2/1
  dotprod2/1 -> Mux/2
  "IW{1,1}(3,:)'"/1 -> dotprod3/1
  dotprod3/1 -> Mux/3
  "IW{1,1}(4,:)'"/1 -> dotprod4/1
  dotprod4/1 -> Mux/4
  "IW{1,1}(5,:)'"/1 -> dotprod5/1
  dotprod5/1 -> Mux/5
  "IW{1,1}(6,:)'"/1 -> dotprod6/1
  dotprod6/1 -> Mux/6
  "IW{1,1}(7,:)'"/1 -> dotprod7/1
  dotprod7/1 -> Mux/7
  "IW{1,1}(8,:)'"/1 -> dotprod8/1
  dotprod8/1 -> Mux/8
  "IW{1,1}(9,:)'"/1 -> dotprod9/1
  dotprod9/1 -> Mux/9
  "IW{1,1}(10,:)'"/1 -> dotprod10/1
  dotprod10/1 -> Mux/10
  Mux/1 -> "iz{1,1}"/1

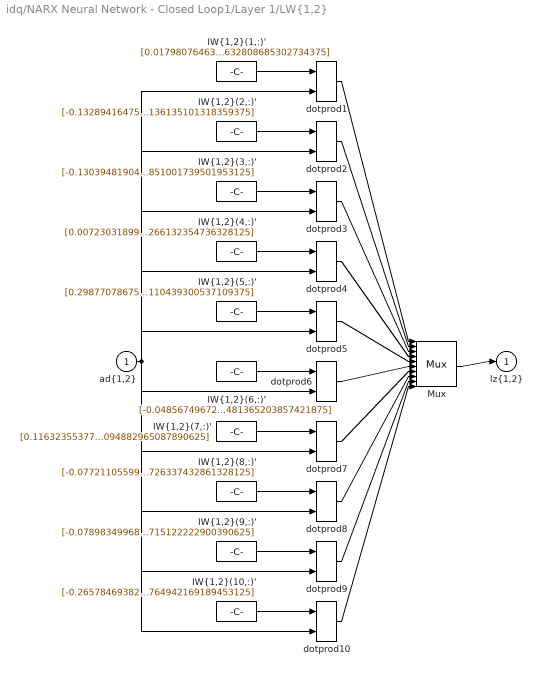
== system idq/NARX Neural Network - Closed Loop1/Layer 1/LW{1,2} ==
  "ad{1,2}" : Inport  PortDimensions=10  SampleTime=1e-05
      mask Display: e = 0.06;c1 = [120 230 180]/255;c2 = ([120 230 180]+0)/(256+128);c3 = ([120 230 180]+128)/(256+128);patch([0 1 1 0],[0 0 1 1],c1);patch([0 1 1 1-e 1-e 0+e],[0 0 1 1-e 0+e 0+e],c2);patch([0 0 1 1-e 0+e 0+e],[0 1 1 1-e 1-e 0+e],c3);plot([0 1 1 0 0],[0 0 1 1 0]);
  "IW{1,2}(1,:)'" : Constant  Value=[0.017980764638247180575714168071499443612992763519287109375;-0.0006884388898641346198059576266814474365673959255218505859375;0.11460027905338464326856495745232678018510341644287109375;0.135802433740163319697558108600787818431854248046875;0.0417070836901971275789691162572125904262065887451171875;0.187143567787656783796279569287435151636600494384765625;0.05116759955733361786567314766216441057622432708740234375;0.13174712189684656404864426804124377667903900146484375;0.109829224742276021498099680684390477836132049560546875;0.09122333474122355789770466572008444927632808685302734375]
      mask Display: e = 0.06;c1 = [120 150 230]/255;c2 = ([120 150 230]+0)/383;c3 = ([120 150 230]+128)/383;patch([0 1 1 0],[0 0 1 1],c1);patch([0 1 1 1-e 1-e 0+e],[0 0 1 1-e 0+e 0+e],c2);patch([0 0 1 1-e 0+e 0+e],[0 1 1 1-e 1-e 0+e],c3);plot([0 1 1 0 0],[0 0 1 1 0]);disp('weights');
  "IW{1,2}(10,:)'" : Constant  Value=[-0.265784693822970485843626420319196768105030059814453125;-0.06802676523812740960739375850607757456600666046142578125;0.2096366117174472964990172840771265327930450439453125;0.2414935230699513379892806597126764245331287384033203125;0.0596576307919906290155864780899719335138797760009765625;0.2040583605379853171513104825862683355808258056640625;0.15905704545408394512406857757014222443103790283203125;0.131804418118469046650176323964842595160007476806640625;0.0786608821238964639466217931840219534933567047119140625;0.09307297361166762261763807373426971025764942169189453125]
      mask Display: e = 0.06;c1 = [120 150 230]/255;c2 = ([120 150 230]+0)/383;c3 = ([120 150 230]+128)/383;patch([0 1 1 0],[0 0 1 1],c1);patch([0 1 1 1-e 1-e 0+e],[0 0 1 1-e 0+e 0+e],c2);patch([0 0 1 1-e 0+e 0+e],[0 1 1 1-e 1-e 0+e],c3);plot([0 1 1 0 0],[0 0 1 1 0]);disp('weights');
  "IW{1,2}(2,:)'" : Constant  Value=[-0.1328941647571120210358230906422249972820281982421875;0.041760579762441608908662971089142956770956516265869140625;0.300977406476627518117084036930464208126068115234375;0.1163565943564725813086369043958256952464580535888671875;-0.135133538483182380485203566422569565474987030029296875;-0.0333122521249077097049706708276062272489070892333984375;0.17687614319344480140472342100110836327075958251953125;0.07608777338393975242514244428093661554157733917236328125;-0.2376845366363752043437074235043837688863277435302734375;0.1128591005765014754214092818074277602136135101318359375]
      mask Display: e = 0.06;c1 = [120 150 230]/255;c2 = ([120 150 230]+0)/383;c3 = ([120 150 230]+128)/383;patch([0 1 1 0],[0 0 1 1],c1);patch([0 1 1 1-e 1-e 0+e],[0 0 1 1-e 0+e 0+e],c2);patch([0 0 1 1-e 0+e 0+e],[0 1 1 1-e 1-e 0+e],c3);plot([0 1 1 0 0],[0 0 1 1 0]);disp('weights');
  "IW{1,2}(3,:)'" : Constant  Value=[-0.130394819045013099501062470153556205332279205322265625;-0.058911588987339780221219598388415761291980743408203125;0.1552891092773753534128644560041720978915691375732421875;0.03923386406291611006036390563167515210807323455810546875;0.039183089224500651515104010513823595829308032989501953125;0.062733761267342369460919826451572589576244354248046875;-0.09111834173013376447780586886437959037721157073974609375;-0.009596242826009397652864407746164943091571331024169921875;-0.00080930608643097769715202272067244848585687577724456787109375;0.0224511326227641479225116682982843485660851001739501953125]
      mask Display: e = 0.06;c1 = [120 150 230]/255;c2 = ([120 150 230]+0)/383;c3 = ([120 150 230]+128)/383;patch([0 1 1 0],[0 0 1 1],c1);patch([0 1 1 1-e 1-e 0+e],[0 0 1 1-e 0+e 0+e],c2);patch([0 0 1 1-e 0+e 0+e],[0 1 1 1-e 1-e 0+e],c3);plot([0 1 1 0 0],[0 0 1 1 0]);disp('weights');
  "IW{1,2}(4,:)'" : Constant  Value=[0.007230318992235625595588199843177790171466767787933349609375;-0.027530049567573565416633840641225106082856655120849609375;0.03931927980824719004449008252777275629341602325439453125;0.1036697490313842340281524911915767006576061248779296875;-0.08800488556615093660440152234514243900775909423828125;-0.0422903883627354648666596403927542269229888916015625;-0.029898614238434172152292234159176587127149105072021484375;-0.04938366367480391538880013513335143215954303741455078125;-0.047652363992253032876078577828593552112579345703125;0.01725052938349276587803871052528847940266132354736328125]
      mask Display: e = 0.06;c1 = [120 150 230]/255;c2 = ([120 150 230]+0)/383;c3 = ([120 150 230]+128)/383;patch([0 1 1 0],[0 0 1 1],c1);patch([0 1 1 1-e 1-e 0+e],[0 0 1 1-e 0+e 0+e],c2);patch([0 0 1 1-e 0+e 0+e],[0 1 1 1-e 1-e 0+e],c3);plot([0 1 1 0 0],[0 0 1 1 0]);disp('weights');
  "IW{1,2}(5,:)'" : Constant  Value=[0.298770786750357952854528775787912309169769287109375;0.1565658388270984302526045439662993885576725006103515625;-0.03629034190341783039368550589642836712300777435302734375;0.02845769943966679205171743660685024224221706390380859375;-0.06332093897910094637548894525025389157235622406005859375;-0.02098231875473570429146974447576212696731090545654296875;0.261792687012228963983062612896901555359363555908203125;-0.2449246884246078781455224770979839377105236053466796875;0.2084687459952666299667356497593573294579982757568359375;-0.1443015658127756173367828296250081621110439300537109375]
      mask Display: e = 0.06;c1 = [120 150 230]/255;c2 = ([120 150 230]+0)/383;c3 = ([120 150 230]+128)/383;patch([0 1 1 0],[0 0 1 1],c1);patch([0 1 1 1-e 1-e 0+e],[0 0 1 1-e 0+e 0+e],c2);patch([0 0 1 1-e 0+e 0+e],[0 1 1 1-e 1-e 0+e],c3);plot([0 1 1 0 0],[0 0 1 1 0]);disp('weights');
  "IW{1,2}(6,:)'" : Constant  Value=[-0.048567496725724357276021692086942493915557861328125;0.049251631944106984140052674092657980509102344512939453125;0.0004353004247698937477506486715128630748949944972991943359375;-0.1621728901973635561528652715423959307372570037841796875;0.155239629465585060597021538342232815921306610107421875;0.043663710965122552731809690840236726216971874237060546875;-0.03155285104801015816367026900479686446487903594970703125;-0.035548053032810687790199466462581767700612545013427734375;0.0575050077603969922446225382373086176812648773193359375;0.027162849826149304544031792829628102481365203857421875]
      mask Display: e = 0.06;c1 = [120 150 230]/255;c2 = ([120 150 230]+0)/383;c3 = ([120 150 230]+128)/383;patch([0 1 1 0],[0 0 1 1],c1);patch([0 1 1 1-e 1-e 0+e],[0 0 1 1-e 0+e 0+e],c2);patch([0 0 1 1-e 0+e 0+e],[0 1 1 1-e 1-e 0+e],c3);plot([0 1 1 0 0],[0 0 1 1 0]);disp('weights');
  "IW{1,2}(7,:)'" : Constant  Value=[0.11632355377996307643773121753838495351374149322509765625;0.02658548085751329115300478633798775263130664825439453125;-0.08825617477343779271325985291696269996464252471923828125;-0.019727139142697337759191356099108816124498844146728515625;-0.059495216370238766800948582158525823615491390228271484375;-0.0342811991043955044400348697308800183236598968505859375;0.0283282351314587503565700643548552761785686016082763671875;-0.0411348273191067814735788488178513944149017333984375;0.026584800562406495083589419436975731514394283294677734375;0.00076116582626404617750726089298041188158094882965087890625]
      mask Display: e = 0.06;c1 = [120 150 230]/255;c2 = ([120 150 230]+0)/383;c3 = ([120 150 230]+128)/383;patch([0 1 1 0],[0 0 1 1],c1);patch([0 1 1 1-e 1-e 0+e],[0 0 1 1-e 0+e 0+e],c2);patch([0 0 1 1-e 0+e 0+e],[0 1 1 1-e 1-e 0+e],c3);plot([0 1 1 0 0],[0 0 1 1 0]);disp('weights');
  "IW{1,2}(8,:)'" : Constant  Value=[-0.0772110559986836919588171213035820983350276947021484375;0.0927026872293682802084191507674404419958591461181640625;-0.041853230921141924836259562425766489468514919281005859375;-0.045658256854441449379411466225064941681921482086181640625;0.027787050178736207028951099573532701469957828521728515625;0.07500594873544452756419786965125240385532379150390625;-0.0193446881333378638279096861651851213537156581878662109375;0.02847460067214689638515068281776621006429195404052734375;-0.01960831834849406651866132733630365692079067230224609375;0.06127345702884086364736759833249379880726337432861328125]
      mask Display: e = 0.06;c1 = [120 150 230]/255;c2 = ([120 150 230]+0)/383;c3 = ([120 150 230]+128)/383;patch([0 1 1 0],[0 0 1 1],c1);patch([0 1 1 1-e 1-e 0+e],[0 0 1 1-e 0+e 0+e],c2);patch([0 0 1 1-e 0+e 0+e],[0 1 1 1-e 1-e 0+e],c3);plot([0 1 1 0 0],[0 0 1 1 0]);disp('weights');
  "IW{1,2}(9,:)'" : Constant  Value=[-0.07898349968991009995011864930347655899822711944580078125;-0.041671010845022164736928260708737070672214031219482421875;0.0963912665178356942163873100071214139461517333984375;-0.004648839649580945553031252615028279251419007778167724609375;0.057964360963715551300357020636511151678860187530517578125;0.078269488635638928553106552499230019748210906982421875;-0.01885610693281325467296483111567795276641845703125;0.00964557155850702396815421479914220981299877166748046875;0.0202762712418979966499943401458949665538966655731201171875;-0.034044424661501350437564639150878065265715122222900390625]
      mask Display: e = 0.06;c1 = [120 150 230]/255;c2 = ([120 150 230]+0)/383;c3 = ([120 150 230]+128)/383;patch([0 1 1 0],[0 0 1 1],c1);patch([0 1 1 1-e 1-e 0+e],[0 0 1 1-e 0+e 0+e],c2);patch([0 0 1 1-e 0+e 0+e],[0 1 1 1-e 1-e 0+e],c3);plot([0 1 1 0 0],[0 0 1 1 0]);disp('weights');
  Mux : Mux  Inputs=10
      mask Display: e = 0.06;c1 = [120 150 230]/255;c2 = ([120 150 230]+0)/383;c3 = ([120 150 230]+128)/383;patch([0 1 1 0],[0 0 1 1],c1);patch([0 1 1 1-e 1-e 0+e],[0 0 1 1-e 0+e 0+e],c2);patch([0 0 1 1-e 0+e 0+e],[0 1 1 1-e 1-e 0+e],c3);plot([0 1 1 0 0],[0 0 1 1 0]);disp('Mux');
  dotprod{1..10} (10 alike) : neural/Weight Functions/dotprod
  "lz{1,2}" : Outport
      mask Display: e = 0.06;c1 = [120 230 180]/255;c2 = ([120 230 180]+0)/(256+128);c3 = ([120 230 180]+128)/(256+128);patch([0 1 1 0],[0 0 1 1],c1);patch([0 1 1 1-e 1-e 0+e],[0 0 1 1-e 0+e 0+e],c2);patch([0 0 1 1-e 0+e 0+e],[0 1 1 1-e 1-e 0+e],c3);plot([0 1 1 0 0],[0 0 1 1 0]);
  wires:
  "IW{1,2}(1,:)'"/1 -> dotprod1/1
  "ad{1,2}"/1 -> dotprod1/2, dotprod2/2, dotprod3/2, dotprod4/2, dotprod5/2, dotprod6/2, dotprod7/2, dotprod8/2, dotprod9/2, dotprod10/2
  dotprod1/1 -> Mux/1
  "IW{1,2}(2,:)'"/1 -> dotprod2/1
  dotprod2/1 -> Mux/2
  "IW{1,2}(3,:)'"/1 -> dotprod3/1
  dotprod3/1 -> Mux/3
  "IW{1,2}(4,:)'"/1 -> dotprod4/1
  dotprod4/1 -> Mux/4
  "IW{1,2}(5,:)'"/1 -> dotprod5/1
  dotprod5/1 -> Mux/5
  "IW{1,2}(6,:)'"/1 -> dotprod6/1
  dotprod6/1 -> Mux/6
  "IW{1,2}(7,:)'"/1 -> dotprod7/1
  dotprod7/1 -> Mux/7
  "IW{1,2}(8,:)'"/1 -> dotprod8/1
  dotprod8/1 -> Mux/8
  "IW{1,2}(9,:)'"/1 -> dotprod9/1
  dotprod9/1 -> Mux/9
  "IW{1,2}(10,:)'"/1 -> dotprod10/1
  dotprod10/1 -> Mux/10
  Mux/1 -> "lz{1,2}"/1
